simulink library "Controller_Lib"  (R2018b)
settings: Solver=VariableStepAuto  StartTime=0.0  StopTime=10.0  RelTol=1e-3
values from neighbouring files (symbols this model uses):
  Damper = 16    [PID_wPlant_Init.m]
  K_d = 50    [PID_wPlant_Init.m]
  K_i = 350    [PID_wPlant_Init.m]
  K_p = 300    [PID_wPlant_Init.m]
  Mass = 10    [PID_wPlant_Init.m]
  Spring = 20    [PID_wPlant_Init.m]
settings Model: Creator=turker.erbasi  LastModifiedBy=turker.erbasi

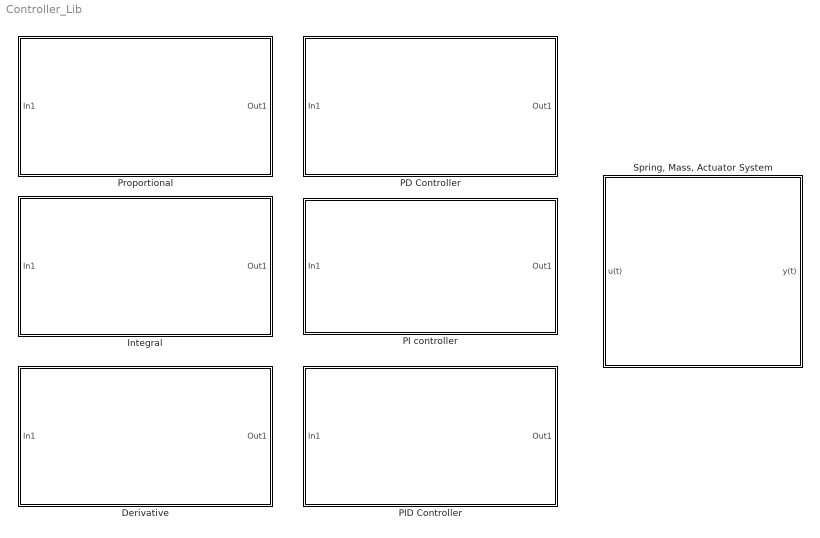
== system Controller_Lib ==
  Derivative : Subsystem
  Integral : Subsystem
  PD Controller : Subsystem
  PI controller : Subsystem
  PID Controller : Subsystem
  Proportional : Subsystem
  "Spring, Mass, Actuator System" : Subsystem

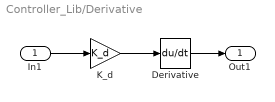
== system Controller_Lib/Derivative ==
  In1 : Inport
  Derivative : Derivative
  K_d : Gain  Gain=K_d
  Out1 : Outport
  wires:
  K_d/1 -> Derivative/1
  Derivative/1 -> Out1/1
  In1/1 -> K_d/1

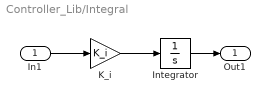
== system Controller_Lib/Integral ==
  In1 : Inport
  Integrator : Integrator
  K_i : Gain  Gain=K_i
  Out1 : Outport
  wires:
  K_i/1 -> Integrator/1
  Integrator/1 -> Out1/1
  In1/1 -> K_i/1

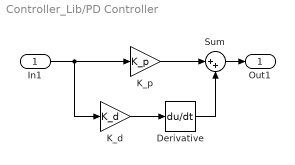
== system Controller_Lib/PD Controller ==
  In1 : Inport
  Derivative : Derivative
  K_d : Gain  Gain=K_d
  K_p : Gain  Gain=K_p
  Sum : Sum  Inputs=|++
  Out1 : Outport
  wires:
  In1/1 -> K_p/1, K_d/1
  Derivative/1 -> Sum/2
  Sum/1 -> Out1/1
  K_p/1 -> Sum/1
  K_d/1 -> Derivative/1

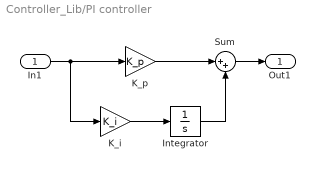
== system Controller_Lib/PI controller ==
  In1 : Inport
  Integrator : Integrator
  K_i : Gain  Gain=K_i
  K_p : Gain  Gain=K_p
  Sum : Sum  Inputs=|++
  Out1 : Outport
  wires:
  K_p/1 -> Sum/1
  Integrator/1 -> Sum/2
  K_i/1 -> Integrator/1
  In1/1 -> K_i/1, K_p/1
  Sum/1 -> Out1/1

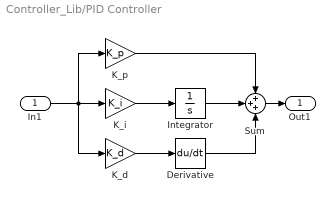
== system Controller_Lib/PID Controller ==
  In1 : Inport
  "Derivative " : Derivative
  Integrator : Integrator
  K_d : Gain  Gain=K_d
  K_i : Gain  Gain=K_i
  K_p : Gain  Gain=K_p
  Sum : Sum  Inputs=+++
  Out1 : Outport
  wires:
  "Derivative "/1 -> Sum/3
  K_p/1 -> Sum/1
  Integrator/1 -> Sum/2
  K_i/1 -> Integrator/1
  In1/1 -> K_i/1, K_d/1, K_p/1
  K_d/1 -> "Derivative "/1
  Sum/1 -> Out1/1

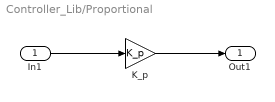
== system Controller_Lib/Proportional ==
  In1 : Inport
  K_p : Gain  Gain=K_p
  Out1 : Outport
  wires:
  In1/1 -> K_p/1
  K_p/1 -> Out1/1

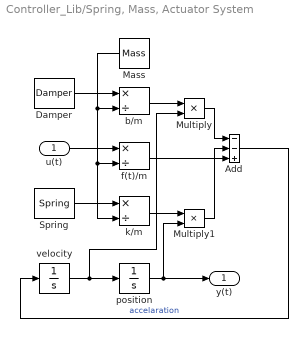
== system Controller_Lib/Spring, Mass, Actuator System ==
  u(t) : Inport
  Add : Sum  Inputs=--+
  Damper : Constant  Value=Damper
  Mass : Constant  Value=Mass
  Multiply : Product
  Multiply1 : Product
  Spring : Constant  Value=Spring
  b/m : Product  Inputs=*/
  f(t)/m : Product  Inputs=*/
  k/m : Product  Inputs=*/
  position : Integrator
  velocity : Integrator
  y(t) : Outport
  wires:
  Multiply1/1 -> Add/2
  Damper/1 -> b/m/1
  Mass/1 -> b/m/2, f(t)/m/2, k/m/2
  Add/1 -> velocity/1  "accelaration"
  position/1 -> y(t)/1, Multiply1/2
  f(t)/m/1 -> Add/3
  k/m/1 -> Multiply1/1
  Multiply/1 -> Add/1
  b/m/1 -> Multiply/1
  velocity/1 -> position/1, Multiply/2
  Spring/1 -> k/m/1
  u(t)/1 -> f(t)/m/1
